simulink model "gm_sampleModel1962_2_sub"  (R2023a)
settings: Solver=VariableStepAuto  StartTime=0.0  StopTime=10.0  RelTol=1e-3
libraries: simulink x3, hdlsllib x1
settings Model: Creator=user1  LastModifiedBy=user1
settings OptimizationCC: BlockReduction=off  ConditionallyExecuteInputs=off
settings DebuggingCC: InheritedTsInSrcMsg=none

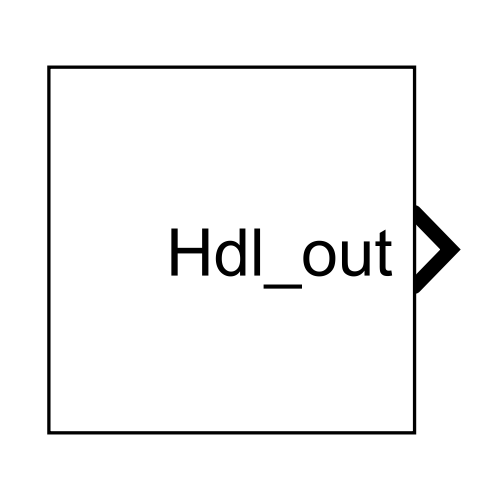
[thumbnail: Simulink's stored preview of the top-level diagram]
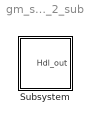
== system gm_sampleModel1962_2_sub ==
  Subsystem : Subsystem

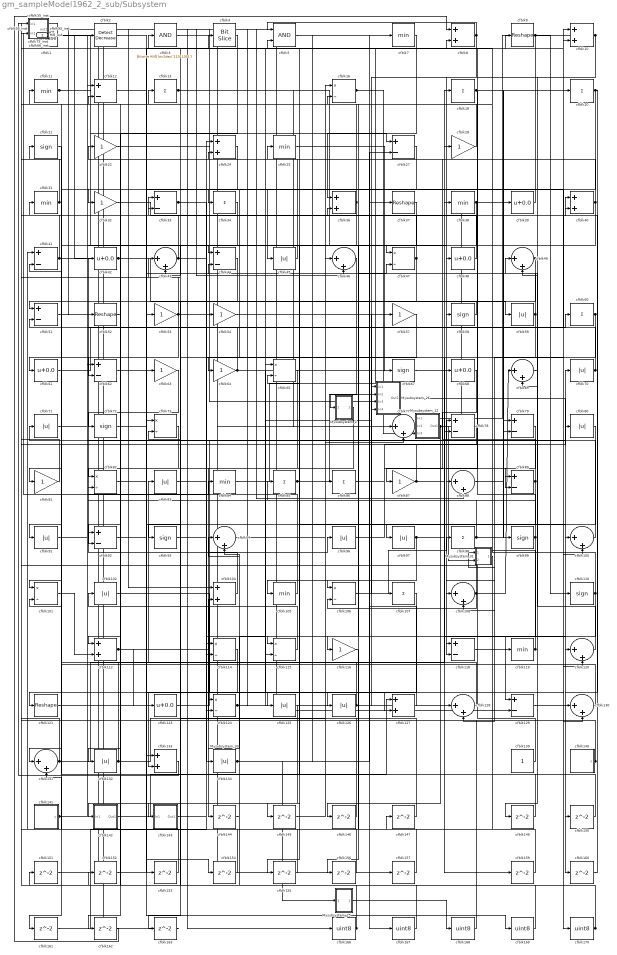
== system gm_sampleModel1962_2_sub/Subsystem ==
  Mysubsystem_12 : Subsystem
  Mysubsystem_2 : Subsystem
  Mysubsystem_25 : Subsystem
  Mysubsystem_26 : Subsystem
  Mysubsystem_31 : Subsystem
  Mysubsystem_33 : Subsystem
  cfblk1 : simulink/Logic and Bit Operations/Detect Increase  vinit=0.0  OutDataTypeStr=uint8
      settings: LibrarySourceBlock=|
      | hdlsllib/Logic and Bit
      | Operations/Detect
      | Increase
  cfblk{8,10,24,36,40,104,112,127,133} (9 alike) : Sum  OutDataTypeStr=uint8
  cfblk{43,46,49,69,77,88,94,100,108,120,128,130..131} (13 alike) : Sum  Inputs=|++  OutDataTypeStr=uint8
  cfblk{16,47,65,73,82,101,106,114..115,124} (10 alike) : Product  Inputs=*/  OutDataTypeStr=uint8  RndMeth=Zero  SaturateOnIntegerOverflow=on
  cfblk{45,59,70..71,80,83,91,96..97,102,125..126,132,134} (14 alike) : Abs  OutDataTypeStr=uint8  SaturateOnIntegerOverflow=off
  cfblk{7,11,25,31,38,84,105,119} (8 alike) : MinMax  OutDataTypeStr=uint8
  cfblk{13,18,20,34,60,85..86,98,107} (9 alike) : Sum  Inputs=+  OutDataTypeStr=uint8
  cfblk{21,58,67,72,93,99,110} (7 alike) : Signum
  cfblk111_inst : Subsystem
  cfblk{22,28,32,53..54,57,63..64,81,87,116} (11 alike) : Gain  OutDataTypeStr=uint8
  cfblk{12,27,33,41,44,51,62,78..79,89,92,118,129} (13 alike) : Sum  Inputs=+-  OutDataTypeStr=uint8
  cfblk{9,37,52,121} (4 alike) : Reshape
  cfblk{39,42,48,61,68,123} (6 alike) : Bias  Bias=0.0  SaturateOnIntegerOverflow=off
  cfblk139 : Constant  OutDataTypeStr=uint8  SampleTime=-1
  cfblk140 : Subsystem  mask(Counter Free-Running){NumBits=double(16), tsamp=double(-1)}
      mask prompts: NumBits "Simulink:masks:NumberOfBits_MP"; tsamp "Simulink:masks:SampleTime_MP"
      mask help: Simulink:masks:CounterFreeRunning_MD
  cfblk141 : Subsystem  mask(Counter Limited){uplimit=double(7), tsamp=double(-1)}
      mask prompts: uplimit "Simulink:masks:UpperLimit_MP"; tsamp "Simulink:masks:SampleTime_MP"
      mask help: Simulink:masks:CounterLimited_MD
      mask init:
      | nbits = double(8);
      | tsamp = double(-1);
      | uplimit = double(7);
  cfblk142 : Subsystem
  cfblk143 : Subsystem
  cfblk{144..147,149..157,159..163} (18 alike) : Delay  SampleTime=1
  cfblk14_inst : Subsystem
  cfblk15_inst : Subsystem
  cfblk{166..170} (5 alike) : DataTypeConversion  OutDataTypeStr=uint8  SaturateOnIntegerOverflow=off  RndMeth=Floor
  cfblk17_inst : Subsystem
  cfblk2 : simulink/Logic and Bit Operations/Detect Decrease  vinit=0.0  OutDataTypeStr=uint8
      settings: LibrarySourceBlock=|
      | hdlsllib/Logic and Bit
      | Operations/Detect
      | Decrease
  cfblk23_inst : Subsystem
  cfblk3 : simulink/Logic and Bit Operations/Bitwise Operator  logicop=AND  UseBitMask=on  BitMask=bin2dec('11011001')  BitMaskRealWorld=Stored Integer
      settings: LibrarySourceBlock=|
      | hdlsllib/Logic and Bit
      | Operations/Bitwise
      | Operator
  cfblk35_inst : Subsystem
  cfblk4 : hdlsllib/Logic and Bit Operations/Bit Slice  lidx=7  ridx=0
  cfblk5 : Logic  AllPortsSameDT=off  OutDataTypeStr=boolean
  cfblk55_inst : Subsystem
  cfblk66_inst : Subsystem
  cfblk75_inst : Subsystem
  cfblk95_inst : Subsystem
  Hdl_out : Outport  OutDataTypeStr=uint8  SampleTime=1
  wires:
  Mysubsystem_12/1(Out1) -> cfblk146/1, Mysubsystem_31/2(In2)
  Mysubsystem_2/1(Out1) -> cfblk144/1
  Mysubsystem_25/1(Out1) -> cfblk168/1
  Mysubsystem_26/1(Out1) -> cfblk160/1
  Mysubsystem_31/1(Out1) -> cfblk147/1
  Mysubsystem_33/1(Out1) -> Mysubsystem_25/1(In1)
  cfblk1/1 -> cfblk44/1
  cfblk10/1 -> cfblk69/2, cfblk118/2, Mysubsystem_12/1(In1)
  cfblk100/1 -> cfblk71/1
  cfblk101/1 -> cfblk112/2
  cfblk102/1 -> cfblk125/1
  cfblk104/1 -> cfblk42/1
  cfblk105/1 -> cfblk14_inst/2(in2)
  cfblk106/1 -> cfblk98/1
  cfblk107/1 -> cfblk133/2
  cfblk108/1 -> cfblk69/1, cfblk106/2, cfblk18/1
  cfblk11/1 -> cfblk27/1, Mysubsystem_33/1(In1)
  cfblk110/1 -> cfblk66_inst/2(in2), cfblk118/1, cfblk115/1
  cfblk111_inst/1(out1) -> cfblk88/2, Mysubsystem_26/3(In3)
  cfblk112/1 -> cfblk96/1, cfblk123/1
  cfblk114/1 -> cfblk121/1
  cfblk115/1 -> cfblk12/2
  cfblk116/1 -> cfblk156/1
  cfblk118/1 -> cfblk129/1
  cfblk119/1 -> cfblk51/2, cfblk13/1
  cfblk12/1 -> cfblk100/1
  cfblk120/1 -> cfblk49/1
  cfblk121/1 -> cfblk53/1
  cfblk123/1 -> cfblk78/1
  cfblk124/1 -> cfblk8/2, Mysubsystem_26/4(In4)
  cfblk125/1 -> cfblk142/1(In1)
  cfblk126/1 -> cfblk83/1, cfblk65/2, cfblk57/1
  cfblk127/1 -> cfblk37/1
  cfblk128/1 -> cfblk11/1
  cfblk129/1 -> cfblk150/1
  cfblk13/1 -> cfblk47/1, Mysubsystem_12/2(In2)
  cfblk130/1 -> cfblk21/1
  cfblk131/1 -> cfblk55_inst/2(in2), cfblk38/1
  cfblk132/1 -> cfblk46/1, cfblk41/2
  cfblk133/1 -> cfblk23_inst/1(in1)
  cfblk134/1 -> cfblk27/2, cfblk7/1
  cfblk139/1 -> cfblk15_inst/1(in1)
  cfblk14_inst/1(out1) -> cfblk129/2
  cfblk140/1(y) -> cfblk104/2, cfblk16/2
  cfblk141/1(y) -> cfblk70/1, cfblk60/1
  cfblk142/1(Out1) -> cfblk127/1
  cfblk143/1(Out1) -> cfblk47/2
  cfblk144/1 -> cfblk94/2
  cfblk145/1 -> cfblk77/2
  cfblk146/1 -> cfblk124/1
  cfblk147/1 -> cfblk73/2
  cfblk149/1 -> cfblk101/2
  cfblk15_inst/1(out1) -> cfblk46/2, cfblk153/1
  cfblk150/1 -> cfblk5/2
  cfblk151/1 -> cfblk133/1
  cfblk152/1 -> cfblk44/2
  cfblk153/1 -> cfblk41/1
  cfblk154/1 -> cfblk17_inst/2(in2)
  cfblk155/1 -> cfblk33/1
  cfblk156/1 -> cfblk131/2
  cfblk157/1 -> cfblk23_inst/2(in2)
  cfblk159/1 -> cfblk36/2
  cfblk16/1 -> Mysubsystem_12/3(In3), cfblk107/1
  cfblk160/1 -> cfblk40/1
  cfblk161/1 -> cfblk114/2
  cfblk162/1 -> cfblk8/1
  cfblk163/1 -> cfblk1/1
  cfblk166/1 -> cfblk94/1, cfblk102/1
  cfblk167/1 -> cfblk75_inst/1(in1)
  cfblk168/1 -> cfblk75_inst/2(in2)
  cfblk169/1 -> cfblk3/1
  cfblk17_inst/1(out1) -> cfblk77/1
  cfblk170/1 -> cfblk152/1, cfblk151/1
  cfblk18/1 -> cfblk79/2, cfblk58/1
  cfblk2/1 -> cfblk34/1
  cfblk20/1 -> cfblk61/1, cfblk130/1, cfblk64/1
  cfblk21/1 -> cfblk91/1
  cfblk22/1 -> cfblk45/1
  cfblk23_inst/1(out1) -> cfblk52/1
  cfblk24/1 -> cfblk101/1
  cfblk25/1 -> cfblk67/1
  cfblk27/1 -> cfblk62/2
  cfblk28/1 -> cfblk66_inst/1(in1)
  cfblk3/1 -> cfblk170/1
  cfblk31/1 -> cfblk95_inst/1(in1), cfblk35_inst/2(in2)
  cfblk32/1 -> cfblk40/2
  cfblk33/1 -> cfblk59/1, cfblk100/2
  cfblk34/1 -> cfblk82/1
  cfblk35_inst/1(out1) -> cfblk68/1
  cfblk36/1 -> cfblk92/2, cfblk33/2, cfblk15_inst/2(in2)
  cfblk37/1 -> cfblk155/1
  cfblk38/1 -> cfblk81/1, cfblk106/1
  cfblk39/1 -> cfblk32/1
  cfblk4/1 -> cfblk72/1
  cfblk40/1 -> cfblk43/2, cfblk22/1
  cfblk41/1 -> cfblk95_inst/2(in2), cfblk48/1, cfblk131/1
  cfblk42/1 -> cfblk114/1, Hdl_out/1
  cfblk43/1 -> cfblk78/2, cfblk126/1, cfblk111_inst/2(in2)
  cfblk44/1 -> cfblk124/2
  cfblk45/1 -> cfblk24/2
  cfblk46/1 -> Mysubsystem_2/1(In1)
  cfblk47/1 -> cfblk93/1, cfblk35_inst/1(in1)
  cfblk48/1 -> cfblk111_inst/1(in1)
  cfblk49/1 -> cfblk116/1, cfblk143/1(In1)
  cfblk5/1 -> cfblk167/1
  cfblk51/1 -> cfblk2/1
  cfblk52/1 -> cfblk132/1
  cfblk53/1 -> cfblk55_inst/1(in1), cfblk120/2, cfblk161/1
  cfblk54/1 -> cfblk99/1
  cfblk55_inst/1(out1) -> cfblk63/1
  cfblk57/1 -> cfblk163/1
  cfblk58/1 -> cfblk51/1
  cfblk59/1 -> cfblk128/2, cfblk108/1, cfblk31/1
  cfblk60/1 -> cfblk108/2, Mysubsystem_31/1(In1)
  cfblk61/1 -> cfblk10/2
  cfblk62/1 -> cfblk154/1
  cfblk63/1 -> cfblk112/1
  cfblk64/1 -> cfblk24/1, cfblk130/2
  cfblk65/1 -> cfblk162/1
  cfblk66_inst/1(out1) -> cfblk128/1, cfblk157/1
  cfblk67/1 -> cfblk119/1
  cfblk68/1 -> cfblk87/1
  cfblk69/1 -> cfblk149/1
  cfblk7/1 -> cfblk36/1
  cfblk70/1 -> cfblk49/2, cfblk43/1, cfblk12/1
  cfblk71/1 -> cfblk62/1
  cfblk72/1 -> cfblk169/1
  cfblk73/1 -> cfblk92/1
  cfblk75_inst/1(out1) -> cfblk166/1
  cfblk77/1 -> cfblk39/1
  cfblk78/1 -> cfblk73/1
  cfblk79/1 -> cfblk89/2
  cfblk8/1 -> cfblk5/1, Mysubsystem_26/1(In1)
  cfblk80/1 -> cfblk145/1
  cfblk81/1 -> cfblk17_inst/1(in1)
  cfblk82/1 -> cfblk127/2
  cfblk83/1 -> cfblk54/1
  cfblk84/1 -> cfblk9/1
  cfblk85/1 -> Mysubsystem_26/2(In2), cfblk86/1
  cfblk86/1 -> cfblk89/1
  cfblk87/1 -> cfblk14_inst/1(in1), cfblk28/1
  cfblk88/1 -> cfblk79/1
  cfblk89/1 -> cfblk97/1, cfblk82/2, cfblk25/1
  cfblk9/1 -> cfblk88/1, cfblk110/1
  cfblk91/1 -> cfblk84/1
  cfblk92/1 -> cfblk10/1
  cfblk93/1 -> cfblk115/2
  cfblk94/1 -> cfblk16/1
  cfblk95_inst/1(out1) -> cfblk104/1
  cfblk96/1 -> cfblk80/1
  cfblk97/1 -> cfblk120/1, cfblk159/1, cfblk105/1
  cfblk98/1 -> cfblk20/1, cfblk85/1
  cfblk99/1 -> cfblk4/1, cfblk134/1, cfblk65/1

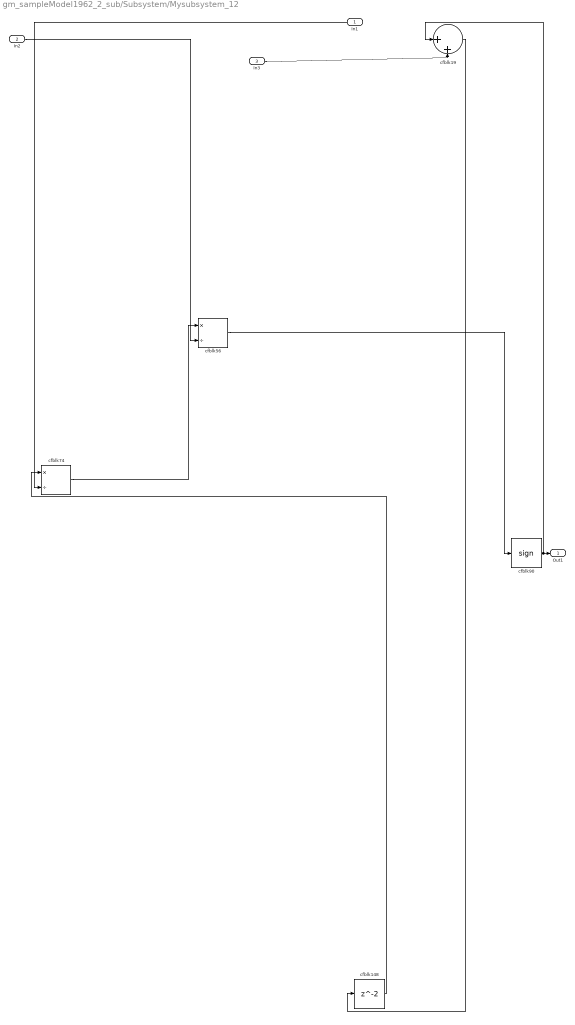
== system gm_sampleModel1962_2_sub/Subsystem/Mysubsystem_12 ==
  In1 : Inport  OutDataTypeStr=uint8  PortDimensions=1  SampleTime=1
  In2 : Inport  Port=2  OutDataTypeStr=uint8  PortDimensions=1  SampleTime=1
  In3 : Inport  Port=3  OutDataTypeStr=uint8  PortDimensions=1  SampleTime=1
  cfblk148 : Delay  SampleTime=1
  cfblk19 : Sum  Inputs=|++
  cfblk56 : Product  Inputs=*/  RndMeth=Zero  SaturateOnIntegerOverflow=on
  cfblk74 : Product  Inputs=*/  RndMeth=Zero  SaturateOnIntegerOverflow=on
  cfblk90 : Signum
  Out1 : Outport  SampleTime=1
  wires:
  In1/1 -> cfblk74/2
  In2/1 -> cfblk56/2
  In3/1 -> cfblk19/2
  cfblk148/1 -> cfblk74/1
  cfblk19/1 -> cfblk148/1
  cfblk56/1 -> cfblk90/1
  cfblk74/1 -> cfblk56/1
  cfblk90/1 -> cfblk19/1, Out1/1

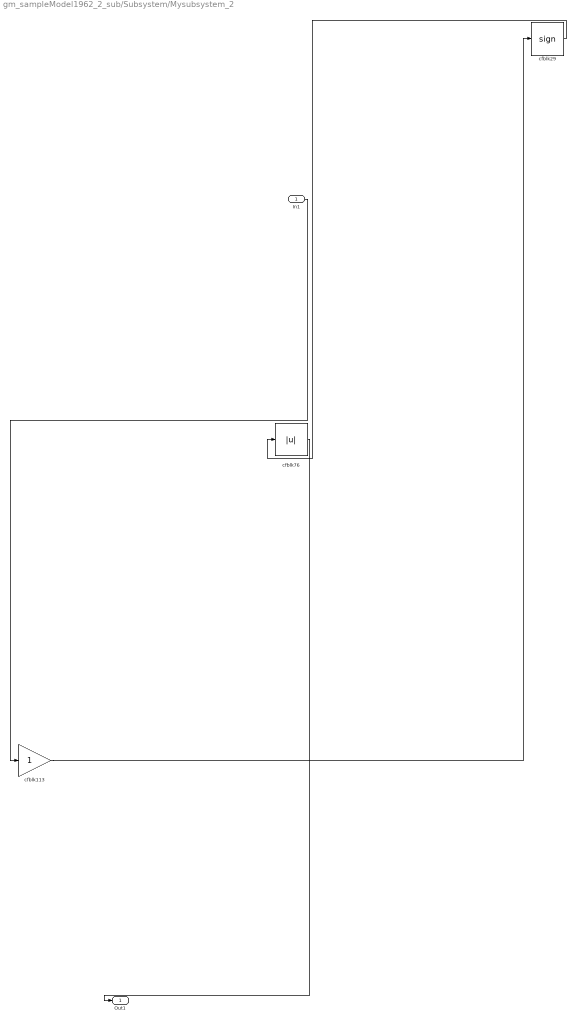
== system gm_sampleModel1962_2_sub/Subsystem/Mysubsystem_2 ==
  In1 : Inport  OutDataTypeStr=uint8  PortDimensions=1  SampleTime=1
  cfblk113 : Gain
  cfblk29 : Signum
  cfblk76 : Abs  SaturateOnIntegerOverflow=off
  Out1 : Outport  SampleTime=1
  wires:
  In1/1 -> cfblk113/1
  cfblk113/1 -> cfblk29/1
  cfblk29/1 -> cfblk76/1
  cfblk76/1 -> Out1/1

== system gm_sampleModel1962_2_sub/Subsystem/Mysubsystem_25 ==
  In1 : Inport  OutDataTypeStr=uint8  PortDimensions=1  SampleTime=1
  cfblk158 : Delay  SampleTime=1
  cfblk164 : DataTypeConversion  OutDataTypeStr=uint8  SaturateOnIntegerOverflow=off  RndMeth=Floor
  Out1 : Outport  SampleTime=1
  wires:
  In1/1 -> cfblk158/1
  cfblk158/1 -> cfblk164/1
  cfblk164/1 -> Out1/1

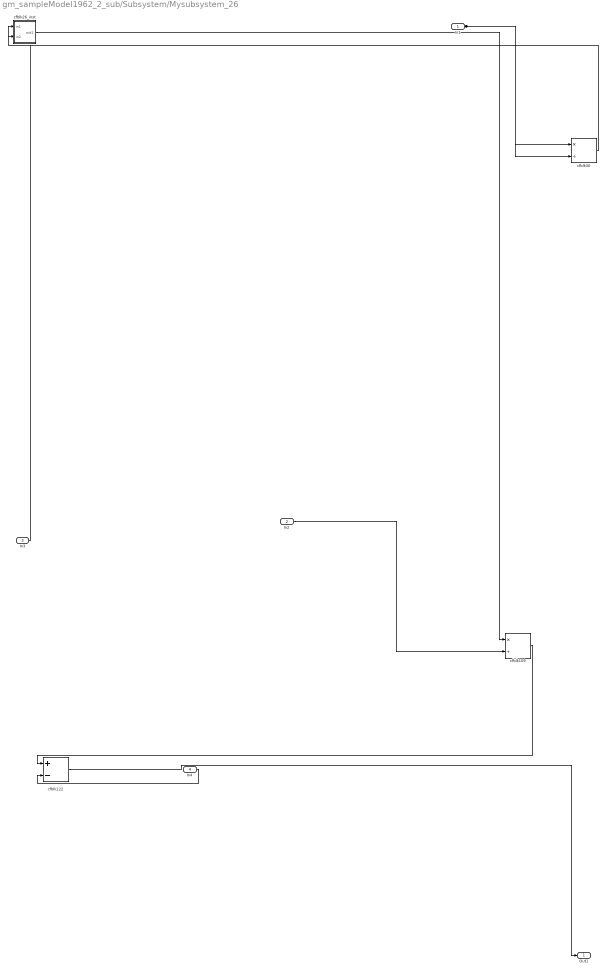
== system gm_sampleModel1962_2_sub/Subsystem/Mysubsystem_26 ==
  In1 : Inport  OutDataTypeStr=uint8  PortDimensions=1  SampleTime=1
  In2 : Inport  Port=2  OutDataTypeStr=uint8  PortDimensions=1  SampleTime=1
  In3 : Inport  Port=3  OutDataTypeStr=uint8  PortDimensions=1  SampleTime=1
  In4 : Inport  Port=4  OutDataTypeStr=uint8  PortDimensions=1  SampleTime=1
  cfblk109 : Product  Inputs=*/  RndMeth=Zero  SaturateOnIntegerOverflow=on
  cfblk122 : Sum  Inputs=+-
  cfblk26_inst : Subsystem
  cfblk30 : Product  Inputs=*/  RndMeth=Zero  SaturateOnIntegerOverflow=on
  Out1 : Outport  SampleTime=1
  wires:
  In1/1 -> cfblk30/2, cfblk30/1
  In2/1 -> cfblk109/2
  In3/1 -> cfblk26_inst/1(in1)
  In4/1 -> cfblk122/2
  cfblk109/1 -> cfblk122/1
  cfblk122/1 -> Out1/1
  cfblk26_inst/1(out1) -> cfblk109/1
  cfblk30/1 -> cfblk26_inst/2(in2)

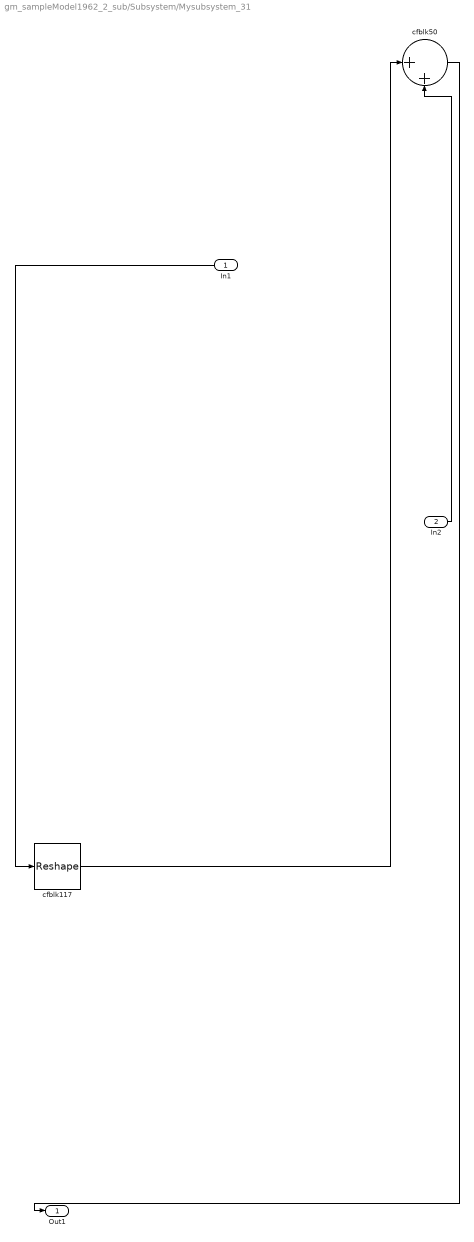
== system gm_sampleModel1962_2_sub/Subsystem/Mysubsystem_31 ==
  In1 : Inport  OutDataTypeStr=uint8  PortDimensions=1  SampleTime=1
  In2 : Inport  Port=2  OutDataTypeStr=uint8  PortDimensions=1  SampleTime=1
  cfblk117 : Reshape
  cfblk50 : Sum  Inputs=|++
  Out1 : Outport  SampleTime=1
  wires:
  In1/1 -> cfblk117/1
  In2/1 -> cfblk50/2
  cfblk117/1 -> cfblk50/1
  cfblk50/1 -> Out1/1

== system gm_sampleModel1962_2_sub/Subsystem/Mysubsystem_33 ==
  In1 : Inport  OutDataTypeStr=uint8  PortDimensions=1  SampleTime=1
  cfblk103 : Bias  Bias=0.0  SaturateOnIntegerOverflow=off
  cfblk165 : DataTypeConversion  OutDataTypeStr=uint8  SaturateOnIntegerOverflow=off  RndMeth=Floor
  Out1 : Outport  SampleTime=1
  wires:
  In1/1 -> cfblk103/1
  cfblk103/1 -> cfblk165/1
  cfblk165/1 -> Out1/1

== system gm_sampleModel1962_2_sub/Subsystem/cfblk111_inst ==
  in1 : Inport  OutDataTypeStr=uint8  SampleTime=1
  in2 : Inport  Port=2  OutDataTypeStr=uint8  SampleTime=1
  mul_cfblk111_dotp_mulcomp : Product  Inputs=**  OutDataTypeStr=uint8  SampleTime=1
  out1 : Outport  OutDataTypeStr=uint8  SampleTime=1
  wires:
  in1/1 -> mul_cfblk111_dotp_mulcomp/1
  in2/1 -> mul_cfblk111_dotp_mulcomp/2
  mul_cfblk111_dotp_mulcomp/1 -> out1/1

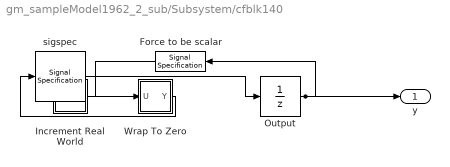
== system gm_sampleModel1962_2_sub/Subsystem/cfblk140 ==
  Force to be scalar : SignalSpecification  DisableCoverage=on  Dimensions=1
  Increment Real World : Subsystem  mask(Real World Value Increment){}
      mask help: Simulink:masks:RealWorldValueIncrement_MD
      mask Display: disp('V++')
  Output : UnitDelay  InitialCondition=0.0  SampleTime=tsamp  HasFrameUpgradeWarning=on
  Wrap To Zero : Subsystem  mask(Wrap To Zero){Threshold=double(65535)}
      mask prompts: Threshold "Simulink:masks:Threshold_MP"
      mask help: Simulink:masks:WrapToZero_MD
  sigspec : SignalSpecification  OutDataTypeStr=uint16  Dimensions=1
  y : Outport  SampleTime=1
  wires:
  Force to be scalar/1 -> Increment Real World/1(u)
  Increment Real World/1(y) -> Wrap To Zero/1(U)
  Output/1 -> Force to be scalar/1, y/1
  Wrap To Zero/1(Y) -> sigspec/1
  sigspec/1 -> Output/1

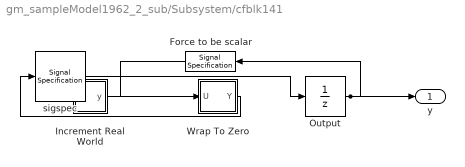
== system gm_sampleModel1962_2_sub/Subsystem/cfblk141 ==
  Force to be scalar : SignalSpecification  DisableCoverage=on  Dimensions=1
  Increment Real World : Subsystem  mask(Real World Value Increment){}
      mask help: Simulink:masks:RealWorldValueIncrement_MD
      mask Display: disp('V++')
  Output : UnitDelay  InitialCondition=0.0  SampleTime=tsamp  HasFrameUpgradeWarning=on
  Wrap To Zero : Subsystem  mask(Wrap To Zero){Threshold=double(7)}
      mask prompts: Threshold "Simulink:masks:Threshold_MP"
      mask help: Simulink:masks:WrapToZero_MD
  sigspec : SignalSpecification  OutDataTypeStr=uint8  Dimensions=1
  y : Outport  SampleTime=1
  wires:
  Force to be scalar/1 -> Increment Real World/1(u)
  Increment Real World/1(y) -> Wrap To Zero/1(U)
  Output/1 -> Force to be scalar/1, y/1
  Wrap To Zero/1(Y) -> sigspec/1
  sigspec/1 -> Output/1

== system gm_sampleModel1962_2_sub/Subsystem/cfblk142 ==
  In1 : Inport  OutDataTypeStr=uint8  PortDimensions=1  SampleTime=1
  Out1 : Outport  SampleTime=1
  wires:
  In1/1 -> Out1/1

== system gm_sampleModel1962_2_sub/Subsystem/cfblk143 ==
  In1 : Inport  OutDataTypeStr=uint8  PortDimensions=1  SampleTime=1
  Out1 : Outport  SampleTime=1
  wires:
  In1/1 -> Out1/1

== system gm_sampleModel1962_2_sub/Subsystem/cfblk14_inst ==
  in1 : Inport  OutDataTypeStr=uint8  SampleTime=1
  in2 : Inport  Port=2  OutDataTypeStr=uint8  SampleTime=1
  mul_cfblk14_dotp_mulcomp : Product  Inputs=**  OutDataTypeStr=uint8  SampleTime=1
  out1 : Outport  OutDataTypeStr=uint8  SampleTime=1
  wires:
  in1/1 -> mul_cfblk14_dotp_mulcomp/1
  in2/1 -> mul_cfblk14_dotp_mulcomp/2
  mul_cfblk14_dotp_mulcomp/1 -> out1/1

== system gm_sampleModel1962_2_sub/Subsystem/cfblk15_inst ==
  in1 : Inport  OutDataTypeStr=uint8  SampleTime=1
  in2 : Inport  Port=2  OutDataTypeStr=uint8  SampleTime=1
  mul_cfblk15_dotp_mulcomp : Product  Inputs=**  OutDataTypeStr=uint8  SampleTime=1
  out1 : Outport  OutDataTypeStr=uint8  SampleTime=1
  wires:
  in1/1 -> mul_cfblk15_dotp_mulcomp/1
  in2/1 -> mul_cfblk15_dotp_mulcomp/2
  mul_cfblk15_dotp_mulcomp/1 -> out1/1

== system gm_sampleModel1962_2_sub/Subsystem/cfblk17_inst ==
  in1 : Inport  OutDataTypeStr=uint8  SampleTime=1
  in2 : Inport  Port=2  OutDataTypeStr=uint8  SampleTime=1
  mul_cfblk17_dotp_mulcomp : Product  Inputs=**  OutDataTypeStr=uint8  SampleTime=1
  out1 : Outport  OutDataTypeStr=uint8  SampleTime=1
  wires:
  in1/1 -> mul_cfblk17_dotp_mulcomp/1
  in2/1 -> mul_cfblk17_dotp_mulcomp/2
  mul_cfblk17_dotp_mulcomp/1 -> out1/1

== system gm_sampleModel1962_2_sub/Subsystem/cfblk23_inst ==
  in1 : Inport  OutDataTypeStr=uint8  SampleTime=1
  in2 : Inport  Port=2  OutDataTypeStr=uint8  SampleTime=1
  mul_cfblk23_dotp_mulcomp : Product  Inputs=**  OutDataTypeStr=uint8  SampleTime=1
  out1 : Outport  OutDataTypeStr=uint8  SampleTime=1
  wires:
  in1/1 -> mul_cfblk23_dotp_mulcomp/1
  in2/1 -> mul_cfblk23_dotp_mulcomp/2
  mul_cfblk23_dotp_mulcomp/1 -> out1/1

== system gm_sampleModel1962_2_sub/Subsystem/cfblk35_inst ==
  in1 : Inport  OutDataTypeStr=uint8  SampleTime=1
  in2 : Inport  Port=2  OutDataTypeStr=uint8  SampleTime=1
  mul_cfblk35_dotp_mulcomp : Product  Inputs=**  OutDataTypeStr=uint8  SampleTime=1
  out1 : Outport  OutDataTypeStr=uint8  SampleTime=1
  wires:
  in1/1 -> mul_cfblk35_dotp_mulcomp/1
  in2/1 -> mul_cfblk35_dotp_mulcomp/2
  mul_cfblk35_dotp_mulcomp/1 -> out1/1

== system gm_sampleModel1962_2_sub/Subsystem/cfblk55_inst ==
  in1 : Inport  OutDataTypeStr=uint8  SampleTime=1
  in2 : Inport  Port=2  OutDataTypeStr=uint8  SampleTime=1
  mul_cfblk55_dotp_mulcomp : Product  Inputs=**  OutDataTypeStr=uint8  SampleTime=1
  out1 : Outport  OutDataTypeStr=uint8  SampleTime=1
  wires:
  in1/1 -> mul_cfblk55_dotp_mulcomp/1
  in2/1 -> mul_cfblk55_dotp_mulcomp/2
  mul_cfblk55_dotp_mulcomp/1 -> out1/1

== system gm_sampleModel1962_2_sub/Subsystem/cfblk66_inst ==
  in1 : Inport  OutDataTypeStr=uint8  SampleTime=1
  in2 : Inport  Port=2  OutDataTypeStr=uint8  SampleTime=1
  mul_cfblk66_dotp_mulcomp : Product  Inputs=**  OutDataTypeStr=uint8  SampleTime=1
  out1 : Outport  OutDataTypeStr=uint8  SampleTime=1
  wires:
  in1/1 -> mul_cfblk66_dotp_mulcomp/1
  in2/1 -> mul_cfblk66_dotp_mulcomp/2
  mul_cfblk66_dotp_mulcomp/1 -> out1/1

== system gm_sampleModel1962_2_sub/Subsystem/cfblk75_inst ==
  in1 : Inport  OutDataTypeStr=uint8  SampleTime=1
  in2 : Inport  Port=2  OutDataTypeStr=uint8  SampleTime=1
  mul_cfblk75_dotp_mulcomp : Product  Inputs=**  OutDataTypeStr=uint8  SampleTime=1
  out1 : Outport  OutDataTypeStr=uint8  SampleTime=1
  wires:
  in1/1 -> mul_cfblk75_dotp_mulcomp/1
  in2/1 -> mul_cfblk75_dotp_mulcomp/2
  mul_cfblk75_dotp_mulcomp/1 -> out1/1

== system gm_sampleModel1962_2_sub/Subsystem/cfblk95_inst ==
  in1 : Inport  OutDataTypeStr=uint8  SampleTime=1
  in2 : Inport  Port=2  OutDataTypeStr=uint8  SampleTime=1
  mul_cfblk95_dotp_mulcomp : Product  Inputs=**  OutDataTypeStr=uint8  SampleTime=1
  out1 : Outport  OutDataTypeStr=uint8  SampleTime=1
  wires:
  in1/1 -> mul_cfblk95_dotp_mulcomp/1
  in2/1 -> mul_cfblk95_dotp_mulcomp/2
  mul_cfblk95_dotp_mulcomp/1 -> out1/1

== system gm_sampleModel1962_2_sub/Subsystem/Mysubsystem_26/cfblk26_inst ==
  in1 : Inport  OutDataTypeStr=uint8  SampleTime=1
  in2 : Inport  Port=2  OutDataTypeStr=uint8  SampleTime=1
  mul_cfblk26_dotp_mulcomp : Product  Inputs=**  OutDataTypeStr=uint16  SampleTime=1
  out1 : Outport  OutDataTypeStr=uint16  SampleTime=1
  wires:
  in1/1 -> mul_cfblk26_dotp_mulcomp/1
  in2/1 -> mul_cfblk26_dotp_mulcomp/2
  mul_cfblk26_dotp_mulcomp/1 -> out1/1

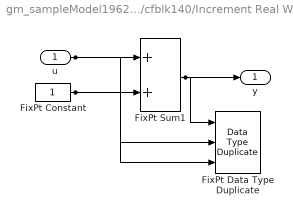
== system gm_sampleModel1962_2_sub/Subsystem/cfblk140/Increment Real World ==
  u : Inport  OutDataTypeStr=uint16  SampleTime=1
  FixPt Constant : Constant  DisableCoverage=on  OutDataTypeStr=Inherit: Inherit via back propagation  SampleTime=-1
  FixPt Data Type Duplicate : DataTypeDuplicate  DisableCoverage=on  NumInputPorts=3
  FixPt Sum1 : Sum  InputSameDT=on  OutDataTypeStr=Inherit: Inherit via back propagation  LockScale=on
  y : Outport  SampleTime=1
  wires:
  u/1 -> FixPt Sum1/1, FixPt Data Type Duplicate/2
  FixPt Constant/1 -> FixPt Sum1/2, FixPt Data Type Duplicate/3
  FixPt Sum1/1 -> FixPt Data Type Duplicate/1, y/1

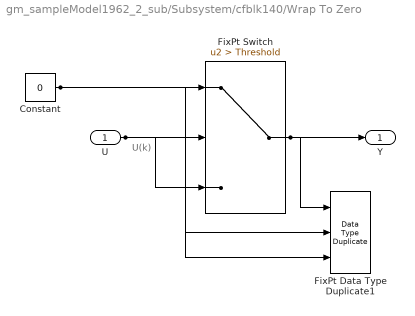
== system gm_sampleModel1962_2_sub/Subsystem/cfblk140/Wrap To Zero ==
  note: U(k)
  U : Inport  OutDataTypeStr=uint16  SampleTime=1
  Constant : Constant  DisableCoverage=on  Value=0  OutDataTypeStr=Inherit: Inherit via back propagation  SampleTime=-1
  FixPt Data Type Duplicate1 : DataTypeDuplicate  DisableCoverage=on  NumInputPorts=3
  FixPt Switch : Switch  Criteria=u2 > Threshold  Threshold=Threshold  OutDataTypeStr=Inherit: Inherit via back propagation  ZeroCross=off  SaturateOnIntegerOverflow=off  InputSameDT=off
  Y : Outport  SampleTime=1
  wires:
  U/1 -> FixPt Switch/3, FixPt Switch/2, FixPt Data Type Duplicate1/2
  Constant/1 -> FixPt Switch/1, FixPt Data Type Duplicate1/3
  FixPt Switch/1 -> FixPt Data Type Duplicate1/1, Y/1

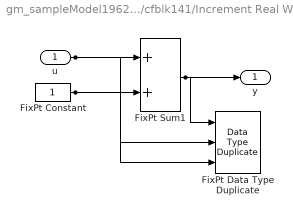
== system gm_sampleModel1962_2_sub/Subsystem/cfblk141/Increment Real World ==
  u : Inport  OutDataTypeStr=uint8  SampleTime=1
  FixPt Constant : Constant  DisableCoverage=on  OutDataTypeStr=Inherit: Inherit via back propagation  SampleTime=-1
  FixPt Data Type Duplicate : DataTypeDuplicate  DisableCoverage=on  NumInputPorts=3
  FixPt Sum1 : Sum  InputSameDT=on  OutDataTypeStr=Inherit: Inherit via back propagation  LockScale=on
  y : Outport  SampleTime=1
  wires:
  u/1 -> FixPt Sum1/1, FixPt Data Type Duplicate/2
  FixPt Constant/1 -> FixPt Sum1/2, FixPt Data Type Duplicate/3
  FixPt Sum1/1 -> FixPt Data Type Duplicate/1, y/1

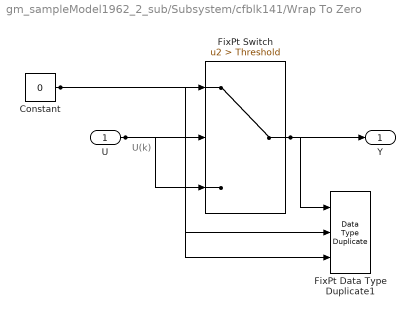
== system gm_sampleModel1962_2_sub/Subsystem/cfblk141/Wrap To Zero ==
  note: U(k)
  U : Inport  OutDataTypeStr=uint8  SampleTime=1
  Constant : Constant  DisableCoverage=on  Value=0  OutDataTypeStr=Inherit: Inherit via back propagation  SampleTime=-1
  FixPt Data Type Duplicate1 : DataTypeDuplicate  DisableCoverage=on  NumInputPorts=3
  FixPt Switch : Switch  Criteria=u2 > Threshold  Threshold=Threshold  OutDataTypeStr=Inherit: Inherit via back propagation  ZeroCross=off  SaturateOnIntegerOverflow=off  InputSameDT=off
  Y : Outport  SampleTime=1
  wires:
  U/1 -> FixPt Switch/3, FixPt Switch/2, FixPt Data Type Duplicate1/2
  Constant/1 -> FixPt Switch/1, FixPt Data Type Duplicate1/3
  FixPt Switch/1 -> FixPt Data Type Duplicate1/1, Y/1
